simulink model "ControlClimatizador"  (R2017a)
settings: Solver=ode45  StartTime=0.0  StopTime=2  RelTol=1e-3  EnableMultiTasking=on
libraries: fuzblock x1
settings Model: Creator=Estela  LastModifiedBy=alexo
settings DataIOCC: LimitDataPoints=on  SaveFormat=Array
settings OptimizationCC: LifeSpan=inf
settings DebuggingCC: SolverPrmCheckMsg=warning  SFUnexpectedBacktrackingDiag=warning  SFNoUnconditionalDefaultTransitionDiag=warning  SFExecutionAtInitializationDiag=none
settings HardwareCC: ProdBitPerPointer=32  ProdBitPerSizeT=32  ProdBitPerPtrDiffT=32  ProdLargestAtomicFloat=None  ProdIntDivRoundTo=Undefined  ProdEndianess=Unspecified  ProdWordSize=32  ProdHWDeviceType=32-bit Generic
settings ModelReferenceCC: PropagateSignalLabelsOutOfModel=off
settings GRTTargetCC: TargetLangStandard=C89/C90 (ANSI)  GeneratePreprocessorConditionals=Disable all
settings ConfigComp: CovMetricSettings=dw  CovHtmlReporting=on  CovSaveCumulativeToWorkspaceVar=on  CovSaveSingleToWorkspaceVar=on  CovExternalEMLEnable=off  CovSFcnEnable=off

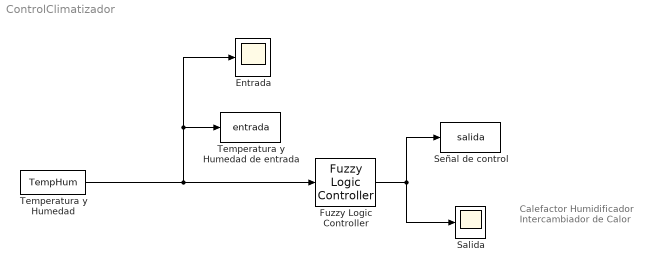
== system ControlClimatizador ==
  note: Calefactor
      | Humidificador
      | Intercambiador de Calor
  Entrada : Scope
  Fuzzy Logic Controller : fuzblock/Fuzzy Logic  Controller  fis='climatizador.fis'
  Salida : Scope
  Señal de control : ToWorkspace  VariableName=salida  SaveFormat=Timeseries  SampleTime=-1
  Temperatura y Humedad : FromWorkspace  VariableName=TempHum  SampleTime=0
  Temperatura y Humedad de entrada : ToWorkspace  VariableName=entrada  SaveFormat=Timeseries  SampleTime=-1
  wires:
  Temperatura y Humedad/1 -> Temperatura y Humedad de entrada/1, Entrada/1, Fuzzy Logic Controller/1
  Fuzzy Logic Controller/1 -> Señal de control/1, Salida/1
